simulink model "Madgwick_embedded"  (R2020a)
settings: Solver=FixedStepDiscrete  StartTime=0.0  StopTime=t(totalNumSamples)  FixedStep=dt  RelTol=1e-3  EnableMultiTasking=on
values from neighbouring files (symbols this model uses):
  beta = sqrt(3/4) * 3.14159265358979 * 5/180    [Madgwick_tests.m]
  dt = 1/fs    (= 0.01)    [Madgwick_tests.m]
libraries: dspmathops x1, aerolibutil x1, robotcorelib x1, aerolibanim x1
settings Model: CodeVerificationMode=processor-in-the-loop (pil)  Creator=wkula  LastModifiedBy=wkula
settings OptimizationCC: DefaultParameterBehavior=Inlined  UseDivisionForNetSlopeComputation=on  GainParamInheritBuiltInType=on  UseFloatMulNetSlope=on  DefaultUnderspecifiedDataType=single  UseSpecifiedMinMax=on  InlineInvariantSignals=on  StrengthReduction=on  PassReuseOutputArgsAs=Individual arguments  ZeroExternalMemoryAtStartup=off  ZeroInternalMemoryAtStartup=off  NoFixptDivByZeroProtection=on  EfficientFloat2IntCast=on  LifeSpan=inf  MaxStackSize=64  OptimizeBlockOrder=speed  OptimizationPriority=Speed  OptimizationCustomize=off  MultiThreadedLoops=on  EfficientTunableParamExpr=on
settings DebuggingCC: ParameterTunabilityLossMsg=error
settings HardwareCC: ProdBitPerPointer=32  ProdBitPerSizeT=32  ProdBitPerPtrDiffT=32  ProdLargestAtomicInteger=Long  ProdLargestAtomicFloat=Double  ProdWordSize=32  ProdHWDeviceType=ARM Compatible->ARM Cortex
settings SFSimCC: MATLABDynamicMemAlloc=off
settings RTWCC: SystemTargetFile=ert.tlc  GenCodeOnly=on  TemplateMakefile=ert_default_tmf  GenerateReport=on  Toolchain=GNU Tools for ARM Embedded Processors  BuildConfiguration=Faster Runs  LaunchReport=on
settings CodeAppCC: ForceParamTrailComments=on  IgnoreCustomStorageClasses=off  OperatorAnnotations=on  SimulinkDataObjDesc=on  SFDataObjDesc=on  InsertBlockDesc=on
settings ERTTargetCC: CombineSignalStateStructs=on  SuppressErrorStatus=on  SupportNonFinite=off  InlinedParameterPlacement=NonHierarchical  ERTCustomFileTemplate=example_file_process.tlc

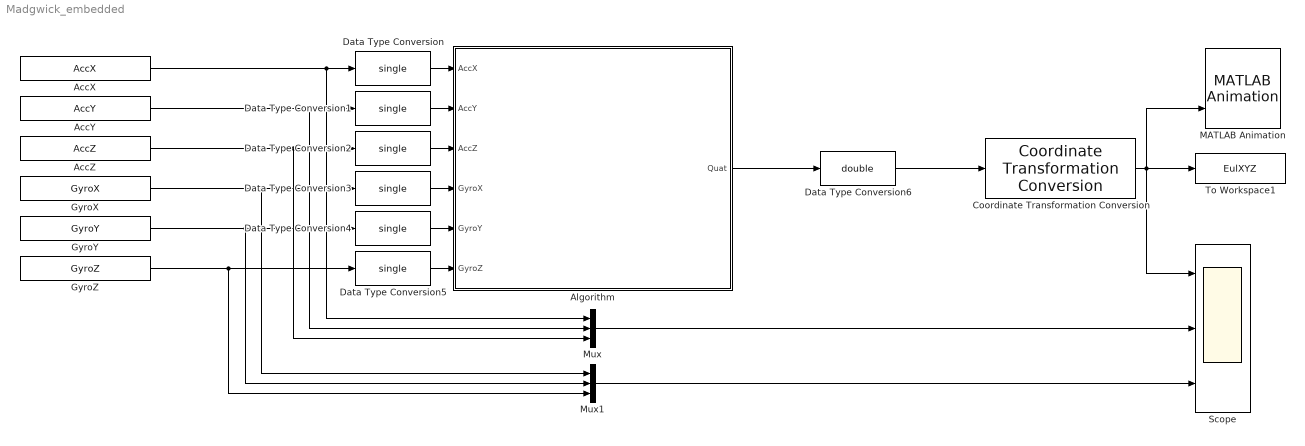
== system Madgwick_embedded ==
  AccX : FromWorkspace  VariableName=AccX  SampleTime=dt
  AccY : FromWorkspace  VariableName=AccY  SampleTime=dt
  AccZ : FromWorkspace  VariableName=AccZ  SampleTime=dt
  Algorithm : Subsystem
  Coordinate Transformation Conversion : robotcorelib/Coordinate Transformation Conversion  InputRepresentation=Quaternion  InputEulerSequence=ZYX  ShowTrVecInputPort=on  OutputRepresentation=Euler Angles  OutputEulerSequence=XYZ  ShowTrVecOutputPort=on  SimulateUsing=Interpreted execution
      settings: SourceProductBaseCode=NV,RO,RR
  Data Type Conversion{,1..5} (6 alike) : DataTypeConversion  OutDataTypeStr=single
  Data Type Conversion6 : DataTypeConversion  OutDataTypeStr=double
  GyroX : FromWorkspace  VariableName=GyroX  SampleTime=dt
  GyroY : FromWorkspace  VariableName=GyroY  SampleTime=dt
  GyroZ : FromWorkspace  VariableName=GyroZ  SampleTime=dt
  MATLAB Animation : aerolibanim/MATLAB Animation  Tag=Matlab Animation 6 DOF  Vehicles=1  Geometries='astredwedge.mat'  BoundingBoxCoordinates=[-50,50,-50,50,-50,50]  CameraOffset=[-150,-50,0]  CameraViewAngle=3  SampleTime=dt  FigurePosition=[962,42,958,981]
      settings: SourceProductBaseCode=AE
  Mux : Mux  Inputs=3
  Mux1 : Mux  Inputs=3
  Scope : Scope  NumInputPorts=3
  To Workspace1 : ToWorkspace  VariableName=EulXYZ  SaveFormat=Timeseries  SampleTime=-1
  wires:
  AccX/1 -> Data Type Conversion/1, Mux/1
  AccY/1 -> Data Type Conversion1/1, Mux/2
  AccZ/1 -> Data Type Conversion2/1, Mux/3
  GyroX/1 -> Data Type Conversion3/1, Mux1/1
  GyroY/1 -> Data Type Conversion4/1, Mux1/2
  GyroZ/1 -> Data Type Conversion5/1, Mux1/3
  Mux/1 -> Scope/2
  Mux1/1 -> Scope/3
  Coordinate Transformation Conversion/1 -> MATLAB Animation/2, To Workspace1/1, Scope/1
  Data Type Conversion/1 -> Algorithm/1(AccX)
  Data Type Conversion1/1 -> Algorithm/2(AccY)
  Data Type Conversion2/1 -> Algorithm/3(AccZ)
  Data Type Conversion3/1 -> Algorithm/4(GyroX)
  Data Type Conversion4/1 -> Algorithm/5(GyroY)
  Data Type Conversion5/1 -> Algorithm/6(GyroZ)
  Algorithm/1(Quat) -> Data Type Conversion6/1
  Data Type Conversion6/1 -> Coordinate Transformation Conversion/1

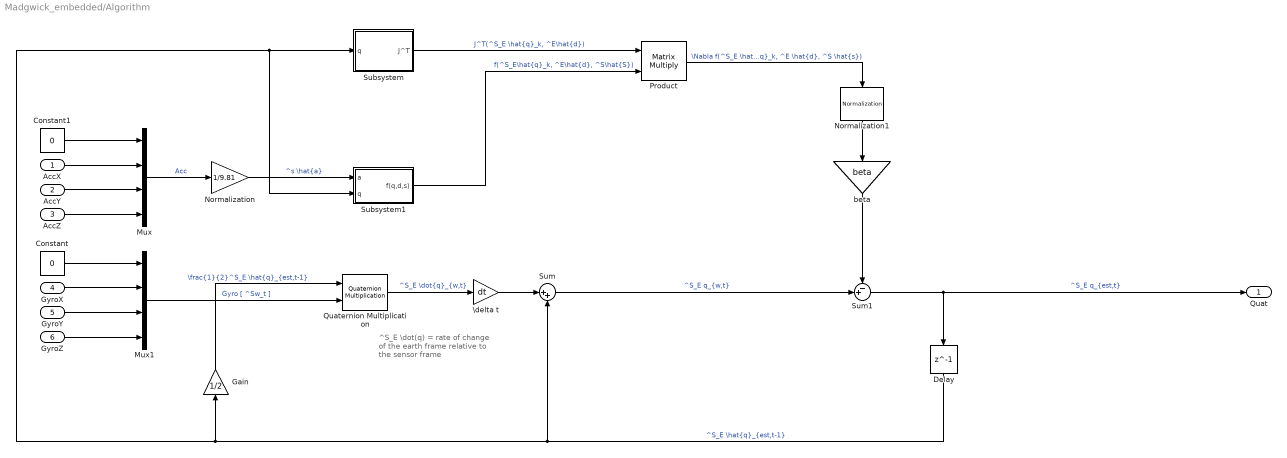
== system Madgwick_embedded/Algorithm ==
  note: ^S_E \dot(q) = rate of change of the earth frame relative to the sensor frame
  AccX : Inport
  AccY : Inport  Port=2
  AccZ : Inport  Port=3
  GyroX : Inport  Port=4
  GyroY : Inport  Port=5
  GyroZ : Inport  Port=6
  Constant : Constant  Value=0  OutDataTypeStr=single
  Constant1 : Constant  Value=0  OutDataTypeStr=single
  Delay : Delay  DelayLength=1  InitialCondition=[1 0 0 0]
  Gain : Gain  Gain=1/2  OutDataTypeStr=Inherit: Same as input
  Mux : Mux
  Mux1 : Mux
  Normalization : Gain  Gain=1/9.81  OutDataTypeStr=Inherit: Same as input  ParamDataTypeStr=Inherit: Same as input
  Normalization1 : dspmathops/Normalization  NormType=2-norm  Bias=1e-10  NormOver=Each column  Dimension=1  roundingMode=Floor  overflowMode=off  outputMin=[]  outputMax=[]
  Product : Product  Multiplication=Matrix(*)  OutDataTypeStr=Inherit: Same as first input
  Quaternion Multiplication : aerolibutil/Quaternion Multiplication
  Subsystem : Subsystem
  Subsystem1 : Subsystem
  Sum : Sum  Inputs=|++  OutDataTypeStr=Inherit: Same as first input
  Sum1 : Sum  Inputs=-+|  AccumDataTypeStr=single  OutDataTypeStr=single
  \delta t : Gain  Gain=dt  OutDataTypeStr=Inherit: Same as input
  beta : Gain  Gain=beta  OutDataTypeStr=Inherit: Same as input  ParamDataTypeStr=Inherit: Same as input
  Quat : Outport
  wires:
  AccY/1 -> Mux/3
  AccX/1 -> Mux/2
  GyroZ/1 -> Mux1/4
  GyroX/1 -> Mux1/2
  AccZ/1 -> Mux/4
  GyroY/1 -> Mux1/3
  Constant/1 -> Mux1/1
  Constant1/1 -> Mux/1
  Gain/1 -> Quaternion Multiplication/1  "\\frac{1}{2}^S_E \\hat{q}_{est,t-1}"
  Quaternion Multiplication/1 -> \delta t/1  "^S_E \\dot{q}_{w,t}"
  Mux1/1 -> Quaternion Multiplication/2  "Gyro [ ^Sw_t ]"
  Delay/1 -> Subsystem1/2(q), Subsystem/1(q), Gain/1, Sum/2  "^S_E \\hat{q}_{est,t-1}"
  \delta t/1 -> Sum/1
  Sum/1 -> Sum1/2  "^S_E q_{w,t}"
  Sum1/1 -> Quat/1, Delay/1  "^S_E q_{est,t}"
  Mux/1 -> Normalization/1  "Acc"
  Subsystem/1(J^T) -> Product/1  "J^T(^S_E \\hat{q}_k, ^E\\hat{d})"
  Subsystem1/1(f(q,d,s)) -> Product/2  "f(^S_E\\hat{q}_k, ^E\\hat{d}, ^S\\hat{S})"
  Product/1 -> Normalization1/1  "\\Nabla f(^S_E \\hat{q}_k, ^E \\hat{d}, ^S \\hat{s})"
  Normalization/1 -> Subsystem1/1(a)  "^s \\hat{a}"
  Normalization1/1 -> beta/1
  beta/1 -> Sum1/1

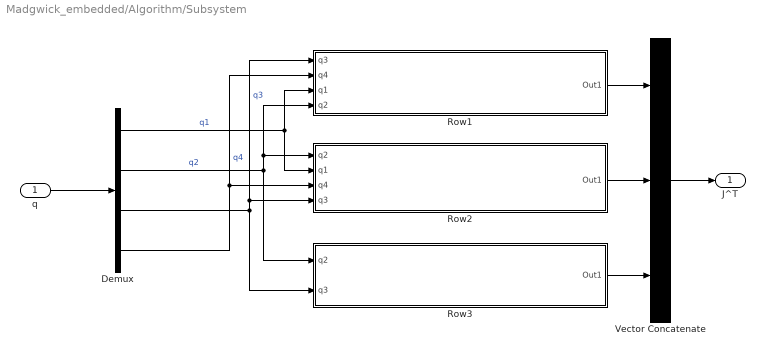
== system Madgwick_embedded/Algorithm/Subsystem ==
  q : Inport
  Demux : Demux
  Row1 : Subsystem
  Row2 : Subsystem
  Row3 : Subsystem
  Vector Concatenate : Concatenate  NumInputs=3  Mode=Multidimensional array  ConcatenateDimension=2
  J^T : Outport
  wires:
  q/1 -> Demux/1
  Demux/1 -> Row2/2(q1), Row1/3(q1)  "q1"
  Demux/2 -> Row3/1(q2), Row1/4(q2), Row2/1(q2)  "q2"
  Demux/3 -> Row3/2(q3), Row1/1(q3), Row2/4(q3)  "q3"
  Demux/4 -> Row1/2(q4), Row2/3(q4)  "q4"
  Vector Concatenate/1 -> J^T/1
  Row1/1(Out1) -> Vector Concatenate/1
  Row2/1(Out1) -> Vector Concatenate/2
  Row3/1(Out1) -> Vector Concatenate/3

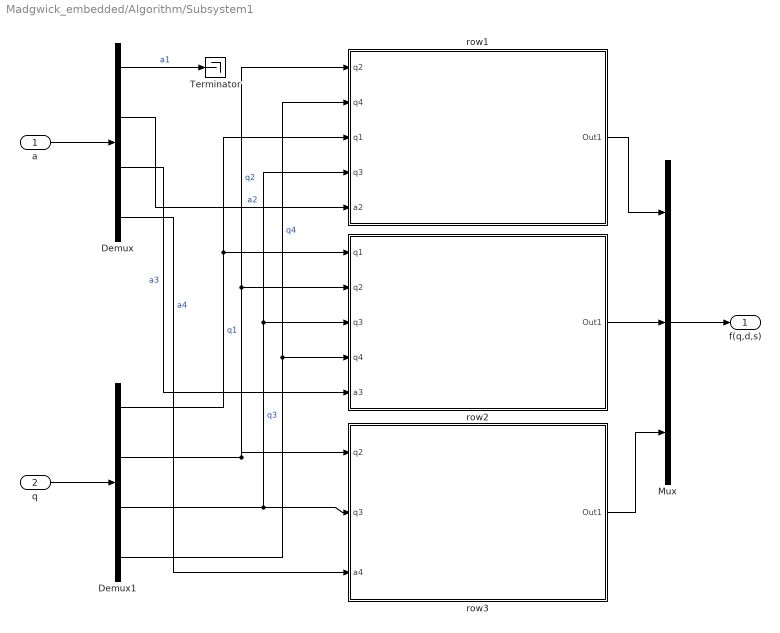
== system Madgwick_embedded/Algorithm/Subsystem1 ==
  a : Inport
  q : Inport  Port=2
  Demux : Demux
  Demux1 : Demux
  Mux : Mux  Inputs=3
  Terminator : Terminator
  row1 : Subsystem
  row2 : Subsystem
  row3 : Subsystem
  f(q,d,s) : Outport
  wires:
  a/1 -> Demux/1
  q/1 -> Demux1/1
  Demux/1 -> Terminator/1  "a1"
  Demux/2 -> row1/5(a2)  "a2"
  Demux/3 -> row2/5(a3)  "a3"
  Demux/4 -> row3/3(a4)  "a4"
  Demux1/1 -> row1/3(q1), row2/1(q1)  "q1"
  Demux1/2 -> row1/1(q2), row2/2(q2), row3/1(q2)  "q2"
  Demux1/3 -> row1/4(q3), row2/3(q3), row3/2(q3)  "q3"
  Demux1/4 -> row1/2(q4), row2/4(q4)  "q4"
  Mux/1 -> f(q,d,s)/1
  row1/1(Out1) -> Mux/1
  row2/1(Out1) -> Mux/2
  row3/1(Out1) -> Mux/3

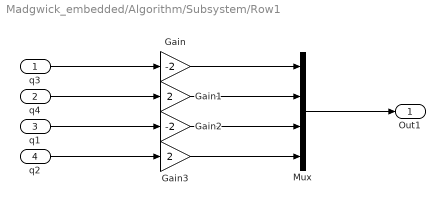
== system Madgwick_embedded/Algorithm/Subsystem/Row1 ==
  q3 : Inport
  q4 : Inport  Port=2
  q1 : Inport  Port=3
  q2 : Inport  Port=4
  Gain : Gain  Gain=-2  ParamDataTypeStr=single  OutDataTypeStr=Inherit: Same as input
  Gain1 : Gain  Gain=2  OutDataTypeStr=single  ParamDataTypeStr=Inherit: Same as input
  Gain2 : Gain  Gain=-2  OutDataTypeStr=single  ParamDataTypeStr=Inherit: Same as input
  Gain3 : Gain  Gain=2  OutDataTypeStr=single  ParamDataTypeStr=Inherit: Same as input
  Mux : Mux
  Out1 : Outport
  wires:
  Mux/1 -> Out1/1
  q3/1 -> Gain/1
  Gain/1 -> Mux/1
  Gain1/1 -> Mux/2
  q4/1 -> Gain1/1
  q1/1 -> Gain2/1
  q2/1 -> Gain3/1
  Gain2/1 -> Mux/3
  Gain3/1 -> Mux/4

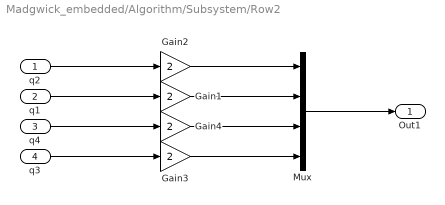
== system Madgwick_embedded/Algorithm/Subsystem/Row2 ==
  q2 : Inport
  q1 : Inport  Port=2
  q4 : Inport  Port=3
  q3 : Inport  Port=4
  Gain{1..4} (4 alike) : Gain  Gain=2  OutDataTypeStr=single  ParamDataTypeStr=Inherit: Same as input
  Mux : Mux
  Out1 : Outport
  wires:
  Gain3/1 -> Mux/4
  Gain4/1 -> Mux/3
  q3/1 -> Gain3/1
  q4/1 -> Gain4/1
  q1/1 -> Gain1/1
  Gain1/1 -> Mux/2
  Gain2/1 -> Mux/1
  q2/1 -> Gain2/1
  Mux/1 -> Out1/1

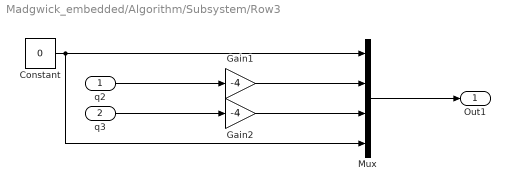
== system Madgwick_embedded/Algorithm/Subsystem/Row3 ==
  q2 : Inport
  q3 : Inport  Port=2
  Constant : Constant  Value=0  OutDataTypeStr=single
  Gain1 : Gain  Gain=-4  OutDataTypeStr=single
  Gain2 : Gain  Gain=-4  OutDataTypeStr=single
  Mux : Mux
  Out1 : Outport
  wires:
  Mux/1 -> Out1/1
  Gain1/1 -> Mux/2
  q2/1 -> Gain1/1
  q3/1 -> Gain2/1
  Gain2/1 -> Mux/3
  Constant/1 -> Mux/4, Mux/1

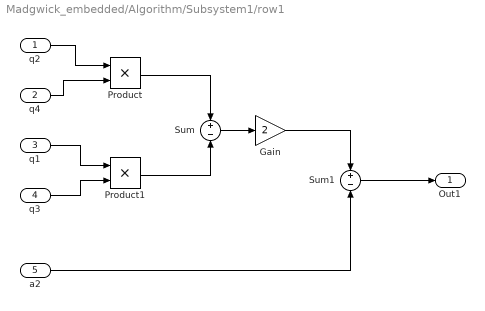
== system Madgwick_embedded/Algorithm/Subsystem1/row1 ==
  q2 : Inport
  q4 : Inport  Port=2
  q1 : Inport  Port=3
  q3 : Inport  Port=4
  a2 : Inport  Port=5
  Gain : Gain  Gain=2  OutDataTypeStr=single  ParamDataTypeStr=Inherit: Same as input
  Product : Product  OutDataTypeStr=Inherit: Same as first input
  Product1 : Product  OutDataTypeStr=Inherit: Same as first input
  Sum : Sum  Inputs=+-  AccumDataTypeStr=single  OutDataTypeStr=single
  Sum1 : Sum  Inputs=+-  AccumDataTypeStr=single  OutDataTypeStr=single
  Out1 : Outport
  wires:
  q2/1 -> Product/1
  q4/1 -> Product/2
  q1/1 -> Product1/1
  q3/1 -> Product1/2
  Product/1 -> Sum/1
  Product1/1 -> Sum/2
  Sum/1 -> Gain/1
  Gain/1 -> Sum1/1
  a2/1 -> Sum1/2
  Sum1/1 -> Out1/1

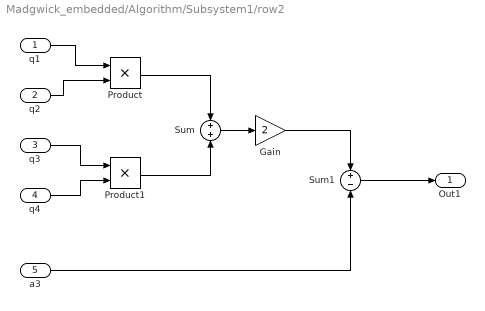
== system Madgwick_embedded/Algorithm/Subsystem1/row2 ==
  q1 : Inport
  q2 : Inport  Port=2
  q3 : Inport  Port=3
  q4 : Inport  Port=4
  a3 : Inport  Port=5
  Gain : Gain  Gain=2  OutDataTypeStr=single  ParamDataTypeStr=Inherit: Same as input
  Product : Product  OutDataTypeStr=Inherit: Same as first input
  Product1 : Product  OutDataTypeStr=Inherit: Same as first input
  Sum : Sum  AccumDataTypeStr=single  OutDataTypeStr=single
  Sum1 : Sum  Inputs=+-  AccumDataTypeStr=single  OutDataTypeStr=single
  Out1 : Outport
  wires:
  Sum1/1 -> Out1/1
  a3/1 -> Sum1/2
  Gain/1 -> Sum1/1
  Sum/1 -> Gain/1
  Product1/1 -> Sum/2
  Product/1 -> Sum/1
  q4/1 -> Product1/2
  q3/1 -> Product1/1
  q2/1 -> Product/2
  q1/1 -> Product/1

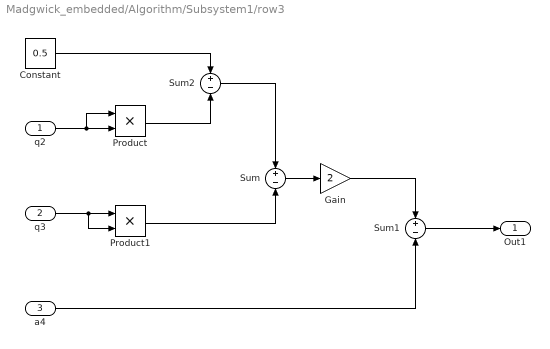
== system Madgwick_embedded/Algorithm/Subsystem1/row3 ==
  q2 : Inport
  q3 : Inport  Port=2
  a4 : Inport  Port=3
  Constant : Constant  Value=0.5  OutDataTypeStr=single
  Gain : Gain  Gain=2  OutDataTypeStr=single  ParamDataTypeStr=Inherit: Same as input
  Product : Product  OutDataTypeStr=Inherit: Same as first input
  Product1 : Product  OutDataTypeStr=Inherit: Same as first input
  Sum : Sum  Inputs=+-  AccumDataTypeStr=single  OutDataTypeStr=single
  Sum1 : Sum  Inputs=+-  AccumDataTypeStr=single  OutDataTypeStr=single
  Sum2 : Sum  Inputs=+-  AccumDataTypeStr=single  OutDataTypeStr=single
  Out1 : Outport
  wires:
  Product1/1 -> Sum/2
  Sum/1 -> Gain/1
  Gain/1 -> Sum1/1
  a4/1 -> Sum1/2
  Sum1/1 -> Out1/1
  q3/1 -> Product1/1, Product1/2
  q2/1 -> Product/1, Product/2
  Constant/1 -> Sum2/1
  Product/1 -> Sum2/2
  Sum2/1 -> Sum/1
